simulink model "Differentiator"  (R2020b)
settings: Solver=VariableStepAuto  StartTime=0.0  StopTime=T  RelTol=1e-3
values from neighbouring files (symbols this model uses):
  A = [0,1;0,0]    [DifferentiatorParameter.m]    (also in PendulumLinearModelTrajectory.m = [0,0,1,0;0,0,0,1;a3;a4])
  alpha = mu_2*C    (= 62.8318530718)    [DifferentiatorParameter.m]    (also in Observer_parameter.m = [alpha_1, 2*alpha_1-1, alpha_2, 2*alpha_2-1]')
  f = 1000    [DifferentiatorParameter.m]
  lambda = mu_1*C^(1/2)    (= 25.0662827463)    [DifferentiatorParameter.m]
  N = 10    [DifferentiatorParameter.m]    (also in PendulumNonLinearModel.m = (pp.p2^2+pp.p3^2)*sin(theta_2)^2+pp.p1*pp.p2-pp.p3^2; PhasePortrait.m = (pp.p2^2+pp.p3^2)*sin(theta_2)^2+pp.p1*pp.p2-pp.p3^2)
  sys_obs = estim(sys,K, 1)    [DifferentiatorParameter.m]
  T = 10    [DifferentiatorParameter.m]    (also in Observer_parameter.m; Project.m)
  Te = 1e-3    (= 0.001)    [DifferentiatorParameter.m]    (also in Observer_parameter.m; Project.m)
libraries: simulink x5, powerlib_meascontrol x1
settings Model: Creator=vorps  LastModifiedBy=vorps
settings SolverCC: ZeroCrossAlgorithm=Adaptive
settings DebuggingCC: IgnoredZcDiagnostic=none

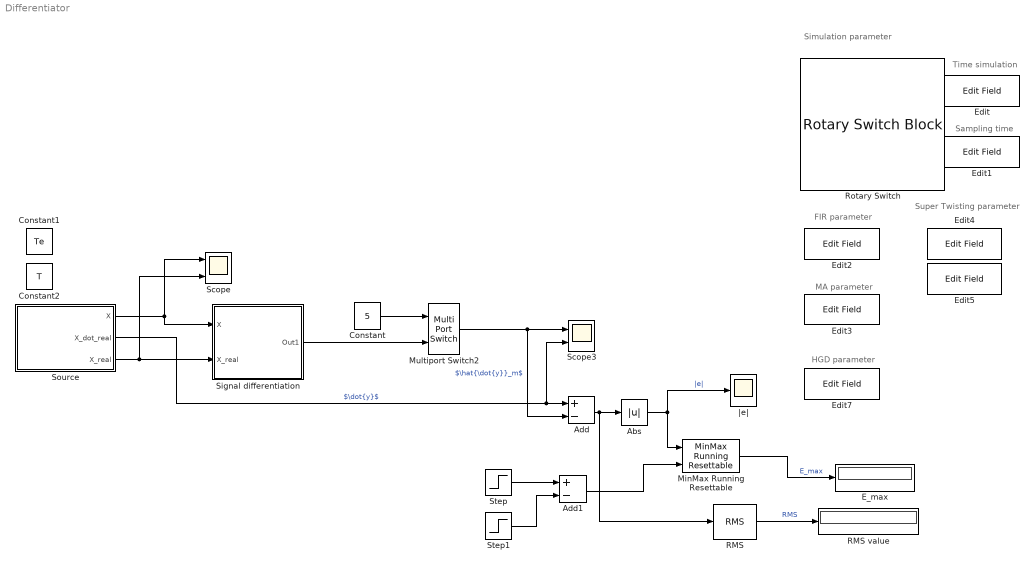
== system Differentiator ==
  note: Simulation parameter
  note: Time simulation
  note: HGD parameter
  note: Super Twisting parameter
  note: Sampling time
  note: FIR parameter
  note: MA parameter
  Abs : Abs  ZeroCross=off
  Add : Sum  Inputs=+-
  Add1 : Sum  Inputs=+-
  Constant : Constant  Value=5
  Constant1 : Constant  Value=Te
  Constant2 : Constant  Value=T
  E_max : Display
  Edit{,1..5,7} (7 alike) : EditField  ShowInitialText=on  Alignment=Left
  MinMax Running Resettable : simulink/Math Operations/MinMax Running Resettable  Function=max  vinit=0.0
  Multiport Switch2 : MultiPortSwitch  Inputs=1
  RMS : powerlib_meascontrol/Measurements/RMS  TrueRMS=off  Freq=1/T  RMSInit=120  Ts=0
  RMS value : Display
  Rotary Switch : RotarySwitchBlock
      settings: Values={{'Real', 'Euler', 'FIR', 'MA', 'Super Twisting', 'HGO'}, [1 2 3 4 5 6]}
  Scope : Scope  NumInputPorts=2
  Scope3 : Scope  NumInputPorts=2
  Signal differentiation : Subsystem
  Source : Subsystem
  Step : Step  Time=0  SampleTime=0
  Step1 : Step  Time=0.5  SampleTime=0
  |e| : Scope
  wires:
  Source/3(X_real) -> Signal differentiation/2(X_real), Scope/2
  Source/2(X_dot_real) -> Scope3/2, Add/1  "$\\dot{y}$"
  Source/1(X) -> Signal differentiation/1(X), Scope/1
  Constant/1 -> Multiport Switch2/1
  Multiport Switch2/1 -> Add/2, Scope3/1  "$\\hat{\\dot{y}}_m$"
  Signal differentiation/1(Out1) -> Multiport Switch2/2
  Add/1 -> RMS/1, Abs/1
  RMS/1 -> RMS value/1  "RMS"
  MinMax Running Resettable/1 -> E_max/1  "E_max"
  Add1/1 -> MinMax Running Resettable/2
  Step/1 -> Add1/1
  Step1/1 -> Add1/2
  Abs/1 -> MinMax Running Resettable/1, |e|/1  "|e|"

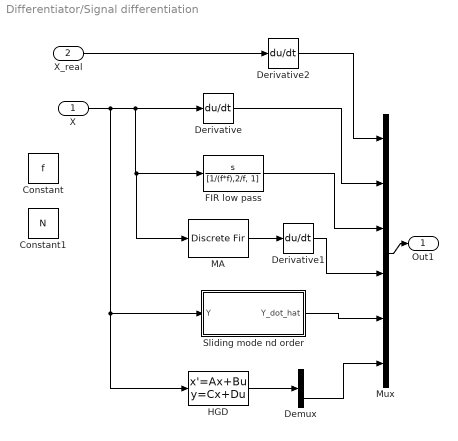
== system Differentiator/Signal differentiation ==
  X : Inport
  X_real : Inport  Port=2
  Constant : Constant  Value=f
  Constant1 : Constant  Value=N
  Demux : Demux  Outputs=3
  Derivative : Derivative  CoefficientInTFapproximation=0
  Derivative1 : Derivative  CoefficientInTFapproximation=0
  Derivative2 : Derivative  CoefficientInTFapproximation=0
  FIR low pass : TransferFcn  Numerator=[1, 0]  Denominator=[1/(f*f),2/f, 1]
  HGD : StateSpace  A=sys_obs.A  B=sys_obs.B  C=sys_obs.C  D=sys_obs.D  InitialCondition=0
  MA : DiscreteFir  Coefficients=1/floor(N)*ones(1,floor(N))  SampleTime=Te
  Mux : Mux  Inputs=6
  Sliding mode nd order : Subsystem
  Out1 : Outport
  wires:
  Derivative/1 -> Mux/2
  FIR low pass/1 -> Mux/3
  Mux/1 -> Out1/1
  MA/1 -> Derivative1/1
  Derivative1/1 -> Mux/4
  X_real/1 -> Derivative2/1
  Derivative2/1 -> Mux/1
  HGD/1 -> Demux/1
  Demux/3 -> Mux/6
  Sliding mode nd order/1(Y_dot_hat) -> Mux/5
  X/1 -> Sliding mode nd order/1(Y), HGD/1, MA/1, FIR low pass/1, Derivative/1

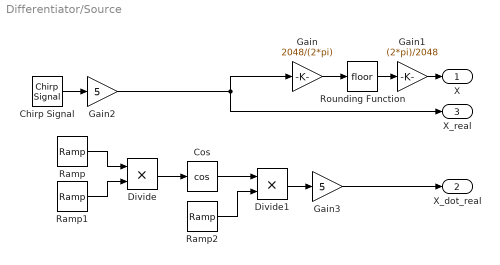
== system Differentiator/Source ==
  Chirp Signal : simulink/Sources/Chirp Signal  f1=0.1  T=T  f2=1
  Cos : Trigonometry  Operator=cos
  Divide : Product  Inputs=**
  Divide1 : Product  Inputs=**
  Gain : Gain  Gain=2048/(2*pi)
  Gain1 : Gain  Gain=(2*pi)/2048
  Gain2 : Gain  Gain=5
  Gain3 : Gain  Gain=5
  Ramp : simulink/Sources/Ramp  slope=2*pi*0.09/2  start=0  InitialOutput=2*pi*0.1
  Ramp1 : simulink/Sources/Ramp  slope=1  start=0  InitialOutput=0
  Ramp2 : simulink/Sources/Ramp  slope=2*pi*0.09  start=0  InitialOutput=2*pi*0.1
  Rounding Function : Rounding
  X : Outport
  X_dot_real : Outport  Port=2
  X_real : Outport  Port=3
  wires:
  Gain/1 -> Rounding Function/1
  Rounding Function/1 -> Gain1/1
  Gain1/1 -> X/1
  Chirp Signal/1 -> Gain2/1
  Gain2/1 -> X_real/1, Gain/1
  Ramp/1 -> Divide/1
  Ramp1/1 -> Divide/2
  Divide1/1 -> Gain3/1
  Ramp2/1 -> Divide1/2
  Divide/1 -> Cos/1
  Cos/1 -> Divide1/1
  Gain3/1 -> X_dot_real/1

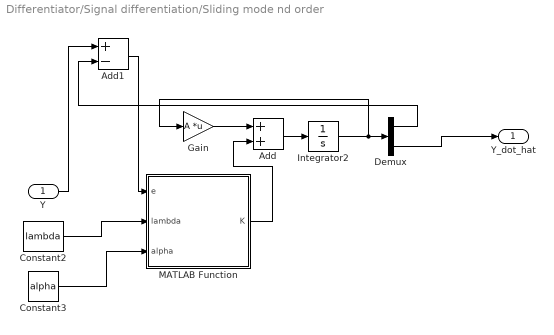
== system Differentiator/Signal differentiation/Sliding mode nd order ==
  Y : Inport
  Add : Sum
  Add1 : Sum  Inputs=+-
  Constant2 : Constant  Value=lambda
  Constant3 : Constant  Value=alpha
  Demux : Demux  Outputs=2
  Gain : Gain  Gain=A  Multiplication=Matrix(K*u)
  Integrator2 : Integrator
  MATLAB Function : MATLAB Function  TreatAsAtomicUnit=on
  Y_dot_hat : Outport
  wires:
  Add/1 -> Integrator2/1
  Gain/1 -> Add/1
  Integrator2/1 -> Demux/1, Gain/1
  Demux/2 -> Y_dot_hat/1
  Demux/1 -> Add1/2
  Y/1 -> Add1/1
  Add1/1 -> MATLAB Function/1(e)
  Constant2/1 -> MATLAB Function/2(lambda)
  Constant3/1 -> MATLAB Function/3(alpha)
  MATLAB Function/1(K) -> Add/2

== matlab function Differentiator/Signal differentiation/Sliding mode nd order/MATLAB Function ==
  data: e input; K output; lambda input; alpha input
function K  = fcn(e, lambda, alpha)
    K = [lambda*abs(e)^(1/2)*sign(e); alpha*sign(e)];
end
